simulink model "FirstPrincInjectorOnly_Testing"  (R2025b)
settings: Solver=VariableStepAuto  StartTime=0.0  StopTime=10.0  RelTol=1e-3
undefined symbols (not defined in the file): A_inj_ox, Cd_inj_ox, epsilon, P_1_ox, P_c_nom, psi_to_Pa, rho_ox
settings Model: Creator=gruby  LastModifiedBy=gruby

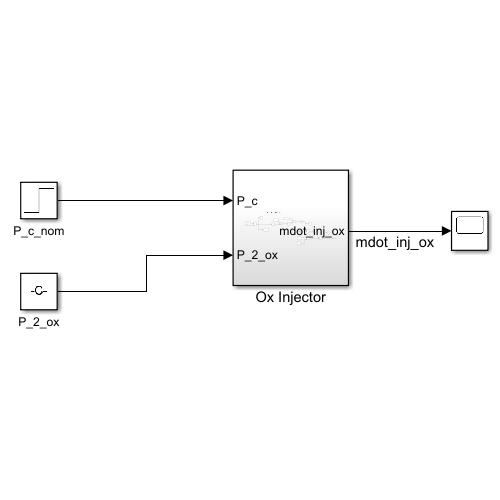
[thumbnail: Simulink's stored preview of the top-level diagram]
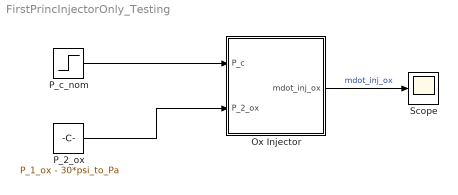
== system FirstPrincInjectorOnly_Testing ==
  Ox Injector : Subsystem
  P_2_ox : Constant  Value=P_1_ox - 30*psi_to_Pa
  P_c_nom : Step  Time=10  Before=P_c_nom  After=P_c_nom  SampleTime=0
  Scope : Scope
  wires:
  P_c_nom/1 -> Ox Injector/1(P_c)
  P_2_ox/1 -> Ox Injector/2(P_2_ox)
  Ox Injector/1(mdot_inj_ox) -> Scope/1  "mdot_inj_ox"

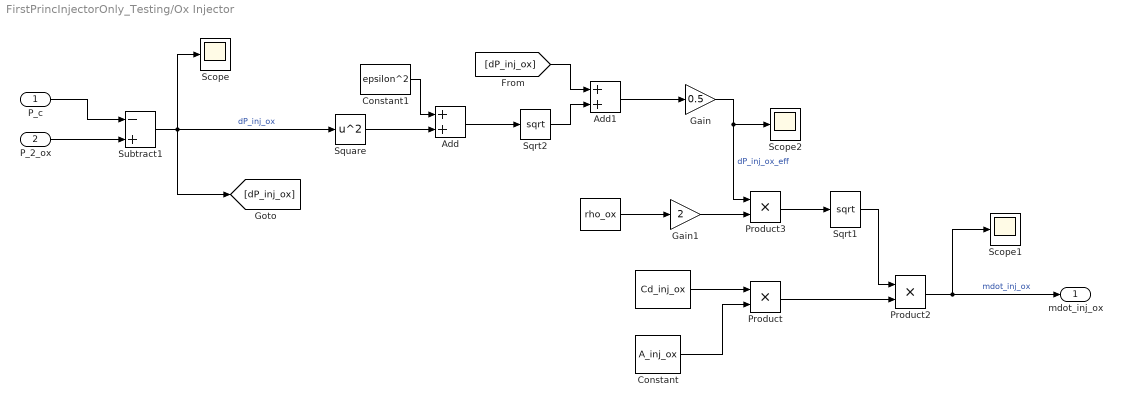
== system FirstPrincInjectorOnly_Testing/Ox Injector ==
  P_c : Inport
  P_2_ox : Inport  Port=2
  " " : Constant  Value=rho_ox
  "    " : Constant  Value=Cd_inj_ox
  Add : Sum
  Add1 : Sum
  Constant : Constant  Value=A_inj_ox
  Constant1 : Constant  Value=epsilon^2
  Gain : Gain  Gain=0.5
  Gain1 : Gain  Gain=2
  Product : Product
  Product2 : Product
  Product3 : Product
  Scope : Scope
      settings: ActiveDisplayYMinimum=-1  ActiveDisplayYMaximum=1
  Scope1 : Scope
      settings: ActiveDisplayYMinimum=0.069456817242045887  ActiveDisplayYMaximum=0.2694568172420459  DataLoggingVariableName=ScopeData2
  Scope2 : Scope
      settings: DataLoggingVariableName=ScopeData21
  Sqrt1 : Sqrt
  Sqrt2 : Sqrt
  Square : Math  Operator=square
  Subtract1 : Sum  Inputs=-+
  mdot_inj_ox : Outport
  wires:
  Subtract1/1 -> [dP_inj_ox], Square/1, Scope/1  "dP_inj_ox"
  "    "/1 -> Product/1
  " "/1 -> Gain1/1
  P_2_ox/1 -> Subtract1/2
  Product3/1 -> Sqrt1/1
  Sqrt1/1 -> Product2/1
  Gain1/1 -> Product3/2
  P_c/1 -> Subtract1/1
  Product2/1 -> Scope1/1, mdot_inj_ox/1  "mdot_inj_ox"
  Constant/1 -> Product/2
  Product/1 -> Product2/2
  Add1/1 -> Gain/1
  Sqrt2/1 -> Add1/2
  Add/1 -> Sqrt2/1
  [dP_inj_ox] -> Add1/1
  Constant1/1 -> Add/1
  Square/1 -> Add/2
  Gain/1 -> Product3/1, Scope2/1  "dP_inj_ox_eff"
